simulink model "submission_without_mask"  (R2021b)
settings: Solver=VariableStepAuto  StartTime=0.0  StopTime=10.0  RelTol=1e-3
undefined symbols (not defined in the file): a, b, cs, css, g, Ib, ks, kss, kt, m1, m2, x0
settings Model: Creator=matth  LastModifiedBy=matth

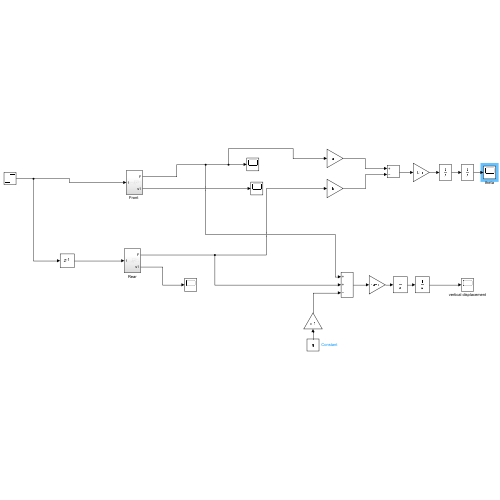
[thumbnail: Simulink's stored preview of the top-level diagram]
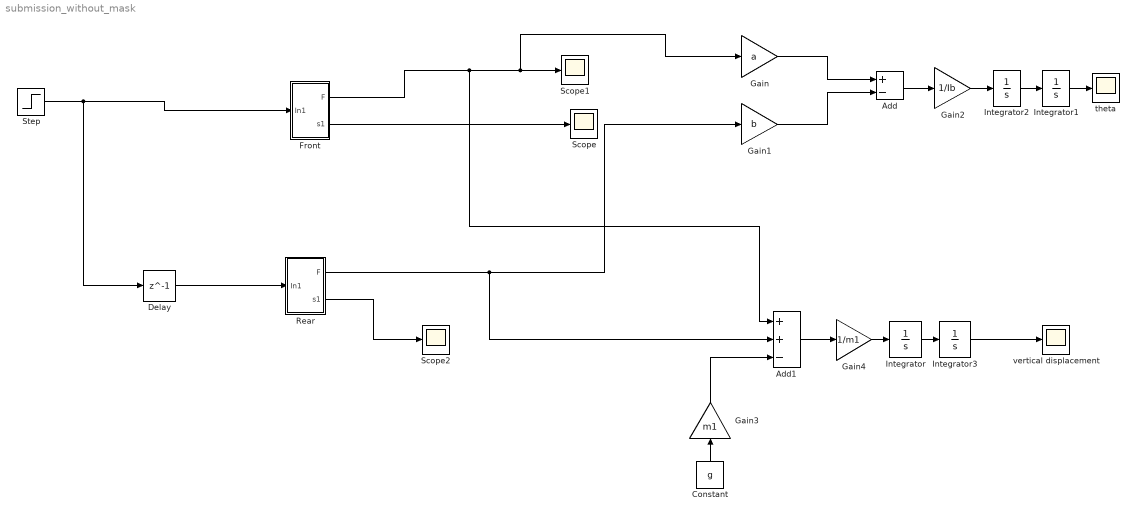
== system submission_without_mask ==
  Add : Sum  Inputs=+-
  Add1 : Sum  Inputs=++-
  Constant : Constant  Value=g
  Delay : Delay  DelayLength=1  InitialCondition=0
  "Front " : Subsystem
  Gain : Gain  Gain=a
  Gain1 : Gain  Gain=b
  Gain2 : Gain  Gain=1/Ib
  Gain3 : Gain  Gain=m1
  Gain4 : Gain  Gain=1/m1
  Integrator{,1..3} (4 alike) : Integrator
  Rear : Subsystem
  Scope : Scope
  Scope1 : Scope
  Scope2 : Scope
  Step : Step  SampleTime=0
  theta : Scope
  vertical displacement : Scope
  wires:
  Step/1 -> Delay/1, "Front "/1(In1)
  "Front "/1(F) -> Add1/1, Gain/1, Scope1/1
  "Front "/2(s1) -> Scope/1
  Delay/1 -> Rear/1(In1)
  Rear/2(s1) -> Scope2/1
  Gain1/1 -> Add/2
  Gain/1 -> Add/1
  Rear/1(F) -> Add1/2, Gain1/1
  Add/1 -> Gain2/1
  Gain2/1 -> Integrator2/1
  Integrator2/1 -> Integrator1/1
  Integrator1/1 -> theta/1
  Constant/1 -> Gain3/1
  Gain3/1 -> Add1/3
  Add1/1 -> Gain4/1
  Gain4/1 -> Integrator/1
  Integrator/1 -> Integrator3/1
  Integrator3/1 -> vertical displacement/1

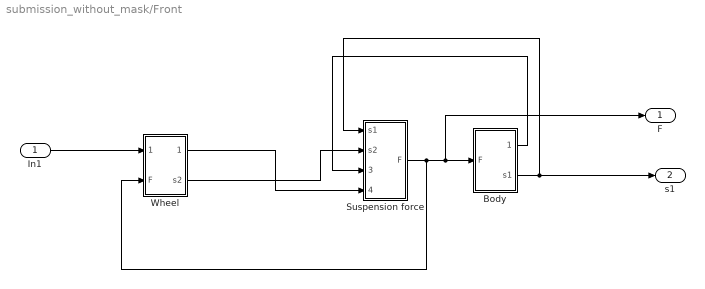
== system submission_without_mask/Front  ==
  In1 : Inport
  Body : Subsystem
  Suspension force : Subsystem
  Wheel : Subsystem
  F : Outport
  s1 : Outport  Port=2
  wires:
  Body/1(S1dot) -> Suspension force/3(S1dot)
  Wheel/2(s2) -> Suspension force/2(s2)
  Body/2(s1) -> s1/1, Suspension force/1(s1)
  Suspension force/1(F) -> Wheel/2(F), F/1, Body/1(F)
  Wheel/1(s2dot) -> Suspension force/4(s2dot)
  In1/1 -> Wheel/1(In1)

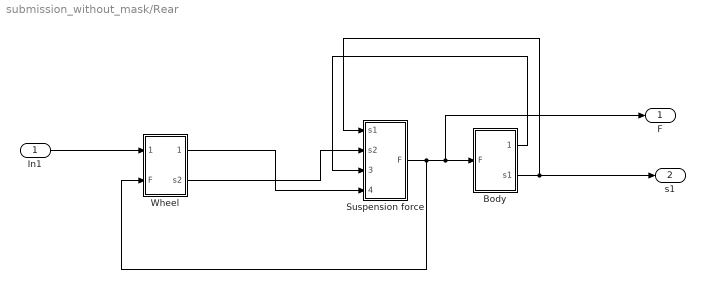
== system submission_without_mask/Rear ==
  In1 : Inport
  Body : Subsystem
  Suspension force : Subsystem
  Wheel : Subsystem
  F : Outport
  s1 : Outport  Port=2
  wires:
  Body/1(S1dot) -> Suspension force/3(S1dot)
  Wheel/2(s2) -> Suspension force/2(s2)
  Body/2(s1) -> s1/1, Suspension force/1(s1)
  Suspension force/1(F) -> Wheel/2(F), F/1, Body/1(F)
  Wheel/1(s2dot) -> Suspension force/4(s2dot)
  In1/1 -> Wheel/1(In1)

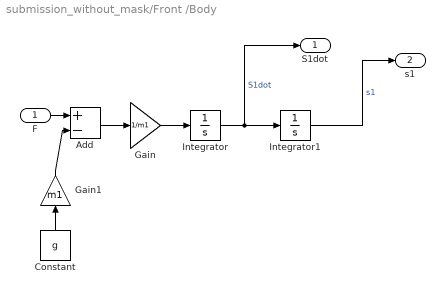
== system submission_without_mask/Front /Body ==
  F : Inport
  Add : Sum  Inputs=+-
  Constant : Constant  Value=g
  Gain : Gain  Gain=1/m1
  Gain1 : Gain  Gain=m1
  Integrator : Integrator
  Integrator1 : Integrator
  S1dot : Outport
  s1 : Outport  Port=2
  wires:
  Gain1/1 -> Add/2
  Add/1 -> Gain/1
  Constant/1 -> Gain1/1
  Gain/1 -> Integrator/1
  Integrator1/1 -> s1/1  "s1"
  Integrator/1 -> S1dot/1, Integrator1/1  "S1dot"
  F/1 -> Add/1

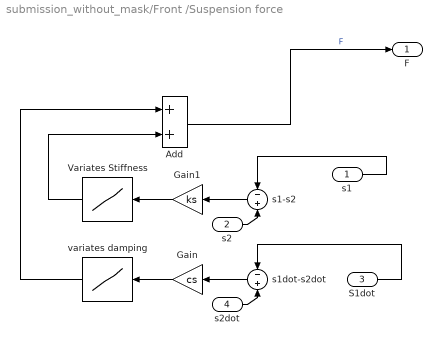
== system submission_without_mask/Front /Suspension force ==
  s1 : Inport
  s2 : Inport  Port=2
  S1dot : Inport  Port=3
  s2dot : Inport  Port=4
  Add : Sum
  Gain : Gain  Gain=cs
  Gain1 : Gain  Gain=ks
  Variates Stiffness : Lookup_n-D  NumberOfTableDimensions=1  BreakpointsForDimension1=[-2*x0, -x0, x0, 2*x0]  Table=[-(ks+kss)*x0, -ks*x0, ks*x0, (ks+kss)*x0]  InternalRulePriority=Speed  RndMeth=Simplest  InputSameDT=on
  s1-s2 : Sum  Inputs=-+
  s1dot-s2dot : Sum  Inputs=-+
  variates damping : Lookup_n-D  NumberOfTableDimensions=1  BreakpointsForDimension1=[-2*x0, -x0, x0, 2*x0]  Table=[-(cs+css)*x0, -cs*x0, cs*x0, (cs+css)*x0]  InternalRulePriority=Speed  RndMeth=Simplest  InputSameDT=on
  F : Outport
  wires:
  Gain1/1 -> Variates Stiffness/1
  variates damping/1 -> Add/1
  S1dot/1 -> s1dot-s2dot/1
  s1dot-s2dot/1 -> Gain/1
  s1-s2/1 -> Gain1/1
  Gain/1 -> variates damping/1
  Add/1 -> F/1  "F"
  Variates Stiffness/1 -> Add/2
  s2dot/1 -> s1dot-s2dot/2
  s1/1 -> s1-s2/1
  s2/1 -> s1-s2/2

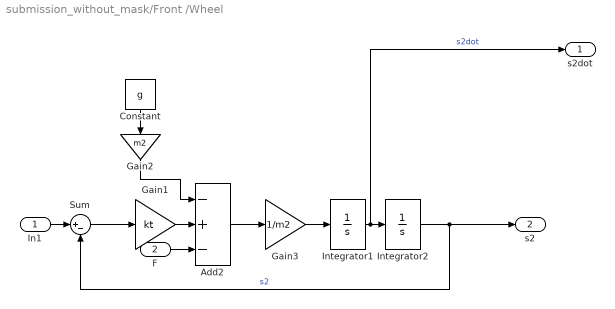
== system submission_without_mask/Front /Wheel ==
  In1 : Inport
  F : Inport  Port=2
  Add2 : Sum  Inputs=-+-
  Constant : Constant  Value=g
  Gain1 : Gain  Gain=kt
  Gain2 : Gain  Gain=m2
  Gain3 : Gain  Gain=1/m2
  Integrator1 : Integrator
  Integrator2 : Integrator
  Sum : Sum  Inputs=|+-
  s2dot : Outport
  s2 : Outport  Port=2
  wires:
  F/1 -> Add2/3
  Gain2/1 -> Add2/1
  Integrator1/1 -> s2dot/1, Integrator2/1  "s2dot"
  Add2/1 -> Gain3/1
  Gain3/1 -> Integrator1/1
  Sum/1 -> Gain1/1
  Gain1/1 -> Add2/2
  Constant/1 -> Gain2/1
  Integrator2/1 -> Sum/2, s2/1  "s2"
  In1/1 -> Sum/1

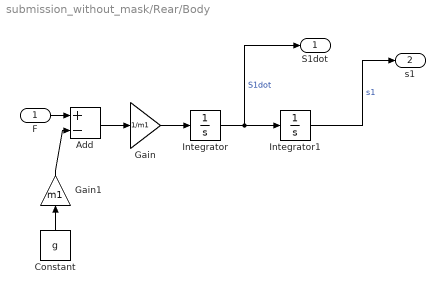
== system submission_without_mask/Rear/Body ==
  F : Inport
  Add : Sum  Inputs=+-
  Constant : Constant  Value=g
  Gain : Gain  Gain=1/m1
  Gain1 : Gain  Gain=m1
  Integrator : Integrator
  Integrator1 : Integrator
  S1dot : Outport
  s1 : Outport  Port=2
  wires:
  Gain1/1 -> Add/2
  Add/1 -> Gain/1
  Constant/1 -> Gain1/1
  Gain/1 -> Integrator/1
  Integrator1/1 -> s1/1  "s1"
  Integrator/1 -> S1dot/1, Integrator1/1  "S1dot"
  F/1 -> Add/1

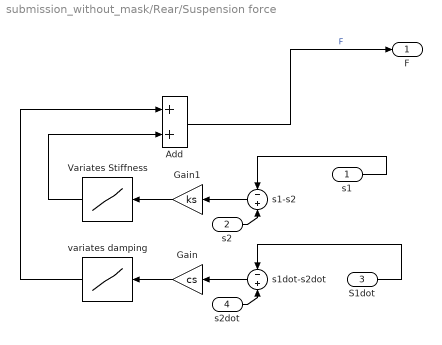
== system submission_without_mask/Rear/Suspension force ==
  s1 : Inport
  s2 : Inport  Port=2
  S1dot : Inport  Port=3
  s2dot : Inport  Port=4
  Add : Sum
  Gain : Gain  Gain=cs
  Gain1 : Gain  Gain=ks
  Variates Stiffness : Lookup_n-D  NumberOfTableDimensions=1  BreakpointsForDimension1=[-2*x0, -x0, x0, 2*x0]  Table=[-(ks+kss)*x0, -ks*x0, ks*x0, (ks+kss)*x0]  InternalRulePriority=Speed  RndMeth=Simplest  InputSameDT=on
  s1-s2 : Sum  Inputs=-+
  s1dot-s2dot : Sum  Inputs=-+
  variates damping : Lookup_n-D  NumberOfTableDimensions=1  BreakpointsForDimension1=[-2*x0, -x0, x0, 2*x0]  Table=[-(cs+css)*x0, -cs*x0, cs*x0, (cs+css)*x0]  InternalRulePriority=Speed  RndMeth=Simplest  InputSameDT=on
  F : Outport
  wires:
  Gain1/1 -> Variates Stiffness/1
  variates damping/1 -> Add/1
  S1dot/1 -> s1dot-s2dot/1
  s1dot-s2dot/1 -> Gain/1
  s1-s2/1 -> Gain1/1
  Gain/1 -> variates damping/1
  Add/1 -> F/1  "F"
  Variates Stiffness/1 -> Add/2
  s2dot/1 -> s1dot-s2dot/2
  s1/1 -> s1-s2/1
  s2/1 -> s1-s2/2

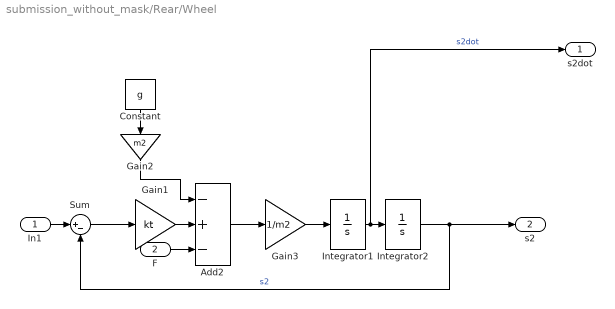
== system submission_without_mask/Rear/Wheel ==
  In1 : Inport
  F : Inport  Port=2
  Add2 : Sum  Inputs=-+-
  Constant : Constant  Value=g
  Gain1 : Gain  Gain=kt
  Gain2 : Gain  Gain=m2
  Gain3 : Gain  Gain=1/m2
  Integrator1 : Integrator
  Integrator2 : Integrator
  Sum : Sum  Inputs=|+-
  s2dot : Outport
  s2 : Outport  Port=2
  wires:
  F/1 -> Add2/3
  Gain2/1 -> Add2/1
  Integrator1/1 -> s2dot/1, Integrator2/1  "s2dot"
  Add2/1 -> Gain3/1
  Gain3/1 -> Integrator1/1
  Sum/1 -> Gain1/1
  Gain1/1 -> Add2/2
  Constant/1 -> Gain2/1
  Integrator2/1 -> Sum/2, s2/1  "s2"
  In1/1 -> Sum/1
